simulink model "mdl_closed_loop_mpc"  (R2023a)
settings: Solver=VariableStepAuto  StartTime=0.0  StopTime=40  RelTol=1e-3
libraries: mpclib x1
settings Model: Creator=hoshino  LastModifiedBy=hoshino
settings ModelReferenceCC: EnableRefExpFcnMdlSchedulingChecks=on

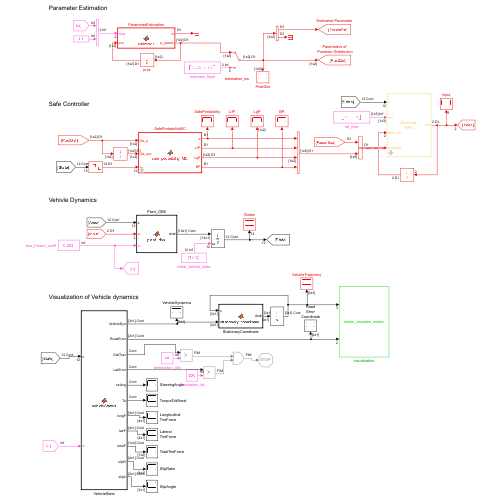
[thumbnail: Simulink's stored preview of the top-level diagram]
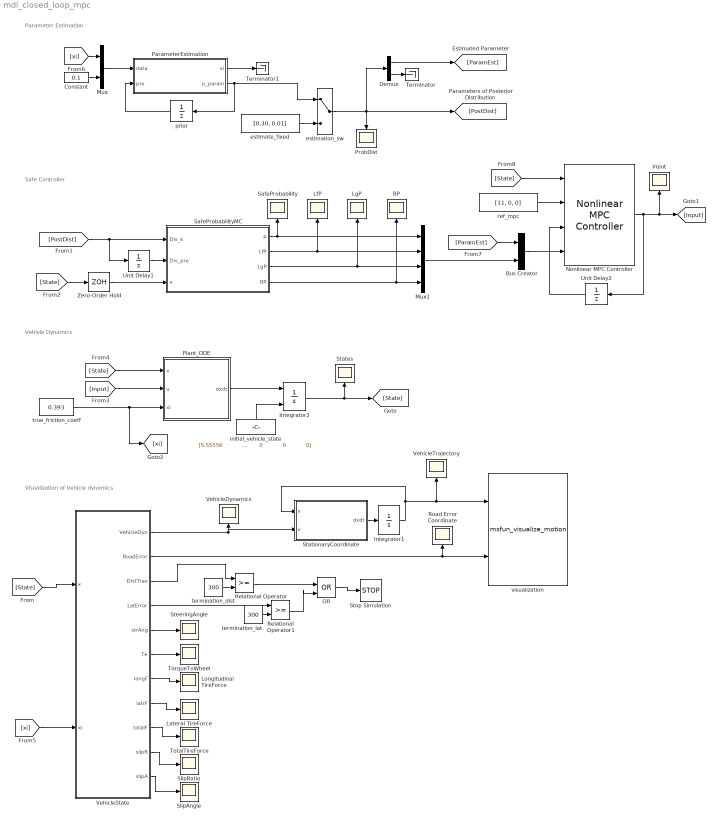
== system mdl_closed_loop_mpc ==
  note: Visualization of Vehicle dynamics
  note: Parameter Estimation
  note: Safe Controller
  note: Vehivle Dynamics
  BP : Scope
  Bus Creator : BusCreator  Inputs=2  OutDataTypeStr=Bus: myBusObject  NonVirtualBus=on
      settings: InheritFromInputs=off
  Constant : Constant  Value=0.1
  Demux : Demux  Outputs=2
  Input : Scope
  Integrator1 : Integrator  InitialCondition=[0; 0; 0]
  Integrator2 : Integrator  InitialConditionSource=external
  Lateral TireForce : Scope
  LfP : Scope
  LgP : Scope
  Longitudinal TireForce : Scope
  Mux : Mux  Inputs=2
  Mux1 : Mux
  Nonlinear MPC Controller : mpclib/Nonlinear MPC Controller  nlmpcobj=nlobj  UseObjectTs=on  UseMEX=off  md_enabled=off  mvtarget_enabled=off  param_enabled=on  cost_enabled=off  mvseq_enabled=off  stateseq_enabled=off  ovseq_enabled=off  slack_enabled=off  status_enabled=off  ov_min=off  ov_max=off  mv_min=off  mv_max=off  mvrate_min=off  mvrate_max=off  state_min=off  state_max=off  ov_weight=off  mv_weight=off  mvrate_weight=off  ecr_weight=off  nlp_initialize=off
  OR : Logic  Operator=OR  IconShape=distinctive  AllPortsSameDT=off  OutDataTypeStr=boolean
  ParameterEstimation : MATLAB Function  TreatAsAtomicUnit=on
  Plant_ODE : MATLAB Function  TreatAsAtomicUnit=on
  ProbDist : Scope
  Relational Operator : RelationalOperator  OutDataTypeStr=boolean  RndMeth=Simplest  InputSameDT=off
  Relational Operator1 : RelationalOperator  OutDataTypeStr=boolean  RndMeth=Simplest  InputSameDT=off
  Road Error Coordinate : Scope
  SafeProbability : Scope
  SafeProbabilityMC : MATLAB Function  TreatAsAtomicUnit=on  mask{snum=100, dt=1.5, horizon=5}
  SlipAngle : Scope
  SlipRatio : Scope
  States : Scope
  StationaryCoordinate : MATLAB Function  TreatAsAtomicUnit=on
  SteeringAngle : Scope
  Stop Simulation : Stop
  Terminator : Terminator
  Terminator1 : Terminator
  TorqueToWheel : Scope
  TotalTireForce : Scope
  Unit Delay1 : UnitDelay  SampleTime=-1  HasFrameUpgradeWarning=on
  Unit Delay2 : UnitDelay  SampleTime=-1  HasFrameUpgradeWarning=on
  VehicleDynamics : Scope
  VehicleState : MATLAB Function  TreatAsAtomicUnit=on
  VehicleTrajectory : Scope
  Zero-Order Hold : ZeroOrderHold  SampleTime=0.1
  estimate_fixed : Constant  Value=[0.30, 0.01]
  estimation_sw : ManualSwitch
  initial_vehicle_state : Constant  Value="[5.55556            0            0            0       17.094       17.094       17.094       17.094            0            0            0            0]"
  prior : UnitDelay  InitialCondition=[0.30, 0.01]  SampleTime=-1  HasFrameUpgradeWarning=on
  ref_mpc : Constant  Value=[11, 0, 0]  VectorParams1D=off
  termination_dist : Constant  Value=300
  termination_lat : Constant  Value=300
  true_friction_coeff : Constant  Value=0.393
  visualization : M-S-Function  FunctionName=msfun_visualize_motion
  wires:
  Integrator2/1 -> States/1, [State]
  VehicleState/1(VehicleDyn) -> StationaryCoordinate/2(v), VehicleDynamics/1
  Integrator1/1 -> VehicleTrajectory/1, visualization/1, StationaryCoordinate/1(x)
  StationaryCoordinate/1(dxdt) -> Integrator1/1
  Plant_ODE/1(dxdt) -> Integrator2/1
  initial_vehicle_state/1 -> Integrator2/2
  true_friction_coeff/1 -> [xi], Plant_ODE/3(xi)
  [State] -> VehicleState/1(x)
  Nonlinear MPC Controller/1 -> Unit Delay2/1, Input/1, [Input]
  ParameterEstimation/2(p_param) -> estimation_sw/1, prior/1
  prior/1 -> ParameterEstimation/2(pre)
  ParameterEstimation/1(xi) -> Terminator1/1
  [State] -> Zero-Order Hold/1
  SafeProbabilityMC/1(p) -> SafeProbability/1, Mux1/1
  Zero-Order Hold/1 -> SafeProbabilityMC/3(x)
  [Input] -> Plant_ODE/2(u)
  [State] -> Plant_ODE/1(x)
  VehicleState/7(longF) -> Longitudinal TireForce/1
  SafeProbabilityMC/4(BP) -> Mux1/4, BP/1
  [PostDist] -> Unit Delay1/1, SafeProbabilityMC/1(Dis_k)
  Unit Delay1/1 -> SafeProbabilityMC/2(Dis_pre)
  VehicleState/9(totalF) -> TotalTireForce/1
  SafeProbabilityMC/2(LfP) -> LfP/1, Mux1/2
  SafeProbabilityMC/3(LgP) -> LgP/1, Mux1/3
  VehicleState/8(latrF) -> Lateral TireForce/1
  [xi] -> VehicleState/2(xi)
  VehicleState/10(slipR) -> SlipRatio/1
  VehicleState/11(slipA) -> SlipAngle/1
  VehicleState/2(RoadError) -> visualization/2, Road Error Coordinate/1
  Mux/1 -> ParameterEstimation/1(data)
  VehicleState/5(strAng) -> SteeringAngle/1
  VehicleState/6(Te) -> TorqueToWheel/1
  Relational Operator/1 -> OR/1
  VehicleState/3(DistTrav) -> Relational Operator/1
  termination_dist/1 -> Relational Operator/2
  estimation_sw/1 -> Demux/1, ProbDist/1, [PostDist]
  estimate_fixed/1 -> estimation_sw/2
  Constant/1 -> Mux/2
  [xi] -> Mux/1
  OR/1 -> Stop Simulation/1
  VehicleState/4(LatError) -> Relational Operator1/1
  termination_lat/1 -> Relational Operator1/2
  Relational Operator1/1 -> OR/2
  Unit Delay2/1 -> Nonlinear MPC Controller/3
  ref_mpc/1 -> Nonlinear MPC Controller/2
  Demux/1 -> [ParamEst]
  Demux/2 -> Terminator/1
  [ParamEst] -> Bus Creator/1
  Bus Creator/1 -> Nonlinear MPC Controller/4
  [State] -> Nonlinear MPC Controller/1
  Mux1/1 -> Bus Creator/2

== matlab function mdl_closed_loop_mpc/StationaryCoordinate ==
  data: x input; v input; dxdt output
function dxdt = stationary_coordinate(x,v)

    % current coordinate
    %X   = x(1); 
    %Y   = x(2); 
    Psi = x(3);
    
    % velocities
    Vx = v(1);
    Vy = v(2);
    r  = v(3);
    
    dxdt = zeros(size(x));
    dxdt(1) = Vx*cos(Psi) - Vy*sin(Psi);
    dxdt(2) = Vy*cos(Psi) + Vx*sin(Psi);
    dxdt(3) = r;

== matlab function mdl_closed_loop_mpc/ParameterEstimation ==
  data: xi output; data input; p_param output; pre input
function [xi, p_param] = estimator(data, pre)

    p_param = mfun_estimator(data, pre);
    xi = p_param(1);

== matlab function mdl_closed_loop_mpc/SafeProbabilityMC ==
  settings: updateMethod=DISCRETE
  data: Dis_k input; Dis_pre input; p output double size=1; x input; dt parameter; snum parameter; horizon parameter; LfP output double size=1; LgP output double size=[1,2]; BP output double size=1
function [p,LfP, LgP, BP] = safe_probability_MC(Dis_k,Dis_pre, x,dt,snum,horizon)

    if Dis_pre == 0
        Dis_pre = Dis_k;
    end
    
    [p, LfP, LgP, BP] = mfun_safe_probability_MC(x, Dis_k,Dis_pre, dt,snum,horizon);

== matlab function mdl_closed_loop_mpc/VehicleState ==
  data: x input; VehicleDyn output; RoadError output; DistTrav output; LatError output; strAng output; Te output; longF output; latrF output; totalF output; xi input; slipR output; slipA output
function [VehicleDyn, RoadError, DistTrav, LatError, strAng, Te, longF, latrF, totalF, slipR, slipA]   = VehicleStates(x, xi)

% Vehicle dyanmics
VehicleDyn = x(1:3);

% Distance traveled
DistTrav = x(10);

% Lateral error
LatError = abs(x(11));


% Road error coordinate
RoadError = x(11:12);

% Steering and Input trque
strAng = x(4);
Te     = x(9);

% Tire forces
tireF = lugre_tireF(x, xi); 
longF = tireF(:,1); % longitudinal force
latrF = tireF(:,2); % lateral force
Ftfl = sqrt( tireF(1,1)^2 + tireF(1,2)^2);
Ftfr = sqrt( tireF(2,1)^2 + tireF(2,2)^2);
Ftrl = sqrt( tireF(3,1)^2 + tireF(3,2)^2);
Ftrr = sqrt( tireF(4,1)^2 + tireF(4,2)^2);
totalF = [Ftfl Ftfr Ftrl Ftrr]; % total force

% Slip ratio and Slip angle
slipR = lugre_slipR(x);
slipA = lugre_slipA(x);

== matlab function mdl_closed_loop_mpc/Plant_ODE ==
  data: x input; u input; dxdt output; xi input
function dxdt = plant_dyn(x,u,xi)

 dxdt = fun_f(x,xi) + fun_g(x)* u;

%   dxdt = suppl_mdl_vehicle_lateral(x,u);
